simulink model "AOO_VOOd1"  (R2025a)
settings: Solver=FixedStepAuto  StartTime=0.0  StopTime=10.0  FixedStep=1e-3  RelTol=1e-3  EnableMultiTasking=on
settings Model: ExtModeTrigDuration=5  Creator=tphil  LastModifiedBy=tphil
settings OptimizationCC: DefaultParameterBehavior=Inlined  EnhancedBackFolding=on  PassReuseOutputArgsAs=Individual arguments  ZeroExternalMemoryAtStartup=off  ZeroInternalMemoryAtStartup=off  MaxStackSize=64  OptimizeBlockOrder=speed  DifferentSizesBufferReuse=on  OptimizationCustomize=off  EfficientTunableParamExpr=on
settings DebuggingCC: ParameterTunabilityLossMsg=error
settings HardwareCC: ProdBitPerPointer=32.0  ProdBitPerSizeT=32.0  ProdBitPerPtrDiffT=32.0  ProdLargestAtomicInteger=Long  ProdLargestAtomicFloat=Double  ProdWordSize=32.0  ProdHWDeviceType=ARM Compatible->ARM Cortex
settings SFSimCC: MATLABDynamicMemAlloc=off
settings RTWCC: SystemTargetFile=ert.tlc  HardwareBoard=NXP FRDM-K64F  TLCOptions="-aInlineSetEventsForThisBaseRateFcn=TLC_FALSE -aSuppressMultiTaskScheduler=TLC_FALSE  -aRateBasedStepFcn=0"  TemplateMakefile=ert_default_tmf  Toolchain=GNU Tools for ARM Embedded Processors  Description=Embedded Coder
settings CodeAppCC: ForceParamTrailComments=on  IgnoreCustomStorageClasses=off  OperatorAnnotations=on  SimulinkDataObjDesc=on  SFDataObjDesc=on  InsertBlockDesc=on
settings ERTTargetCC: ExtModeTransport=4.0  ExtModeStaticAlloc=off  ExtModeMexFile=sendToCommService  ExtModeIntrfLevel=Level1

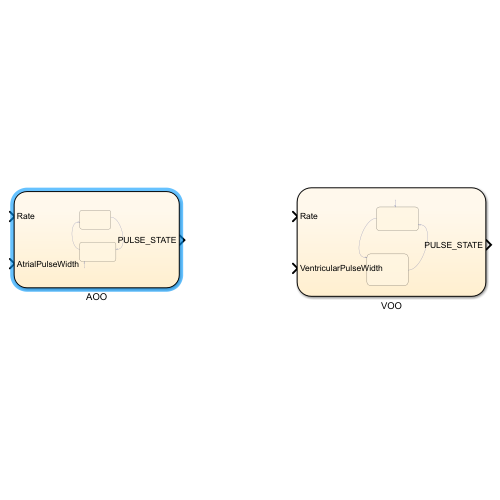
[thumbnail: Simulink's stored preview of the top-level diagram]
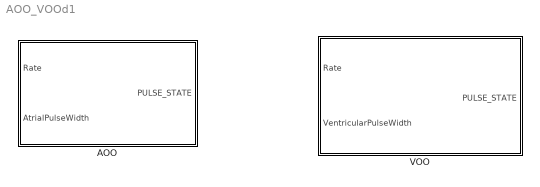
== system AOO_VOOd1 ==
  AOO : Stateflow chart  TreatAsAtomicUnit=on
  VOO : Stateflow chart  TreatAsAtomicUnit=on

== stateflow chart AOO_VOOd1/VOO ==
  state TIMING
    entry:
    PULSE_STATE=false
  state PULSE
    entry:
    PULSE_STATE=true
  (default) -> TIMING
  TIMING -> PULSE : after(120/Rate - VentricularPulseWidth, msec)
  PULSE -> TIMING : after(VentricularPulseWidth, msec)
  data: Rate input int16; VentricularPulseWidth input int16; PULSE_STATE output

== stateflow chart AOO_VOOd1/AOO ==
  state PULSE
    entry:
    PULSE_STATE=true
  state TIMING
    entry:
    PULSE_STATE=false
  PULSE -> TIMING : after(AtrialPulseWidth, msec)
  TIMING -> PULSE : after((120/Rate - AtrialPulseWidth), msec)
  (default) -> TIMING
  data: Rate input int16; AtrialPulseWidth input int16; PULSE_STATE output
